simulink model "MinSeg_Controller"  (R2014b)
settings: Solver=FixedStepDiscrete  SolverMode=SingleTasking  StartTime=0.0  StopTime=inf  FixedStep=TS  RelTol=1e-3
PostLoadFcn:
  | clc
  | 
  | fprintf('Loading MinSegConfigSet...\n')
  | load('MinSegConfig');
  | 
  | fprintf('Attaching MinSegConfigSet...\n')
  | try % Will error if already attached
  | MinSegConfigSet.Name = 'MinSegConfigSet';
  | attachConfigSet('MinSeg_Controller',MinSegConfigSet,false);
  | end
  | 
  | fprintf('Activating MinSegConfigSet...\n')
  | setActiveConfigSet('MinSeg_Controller','MinSegConfigSet');
  | 
  | fprintf('Loading Parameters...\n')
  | MinSeg_Parameters;
  | 
  | fprintf('Model setup complete.\n')
values from neighbouring files (symbols this model uses):
  ES = -C2DEG*D2R    (= -0.00872664625997)    [MinSeg_Parameters.m]    (also in MinSeg_Parameters_v2.m; MinSeg_Parameters_v3.m)
  GS = GyroS*D2R    (= 0.000155832968928)    [MinSeg_Parameters.m]    (also in MinSeg_Parameters_v2.m; MinSeg_Parameters_v3.m)
  Ki = 1*[-r_w -r_w*0 1 1*0]    [MinSeg_Parameters.m]    (also in MinSeg_Parameters_v2.m; MinSeg_Parameters_v3.m)
  KLQRC = KLQR.*[-r_w -r_w 1 1]    [MinSeg_Parameters.m]    (also in MinSeg_Parameters_v2.m; MinSeg_Parameters_v3.m)
  TS = .03    (= 0.03)    [MinSeg_Parameters.m]    (also in MinSeg_Parameters_v2.m = 0.005; MinSeg_Parameters_v3.m = 0.005)
  tstart = 2    [MinSeg_Parameters.m]    (also in MinSeg_Parameters_v2.m; MinSeg_Parameters_v3.m)
  V2DCB = 1/DCB2V    (= 42.5)    [MinSeg_Parameters.m]    (also in MinSeg_Parameters_v2.m = 28.3333333333; MinSeg_Parameters_v3.m = 28.3333333333)
undefined symbols (not defined in the file or in its folder): K
libraries: simulink x4, arduinolib x3, powerlib_meascontrol x1
settings Model: SimulationMode=external  ExtModeTrigDuration=2  Creator=hrlin  LastModifiedBy=mo114c
settings OptimizationCC: ExpressionDepthLimit=2147483647  OptimizeModelRefInitCode=on  LifeSpan=1
settings DebuggingCC: UnderspecifiedInitializationDetection=Classic  MergeDetectMultiDrivingBlocksExec=none  SolverPrmCheckMsg=none  StateNameClashWarn=warning
settings HardwareCC: ProdBitPerInt=16  ProdBitPerPointer=8  ProdIntDivRoundTo=Zero  ProdEndianess=LittleEndian  ProdWordSize=8  ProdHWDeviceType=Atmel->AVR
settings RTWCC: SystemTargetFile=realtime.tlc  GenerateMakefile=off  TemplateMakefile=realtime.tmf  Description=Real-Time Toolbox  RTWVerbose=off  ProcessScript=realtime_make_rtw_hook
settings CodeAppCC: CustomSymbolStrType=$N$R$M  InternalIdentifier=Classic
settings STFCustomTargetCC: TargetLibSuffix=.a  GenerateSampleERTMain=on  ERTCustomFileBanners=on  SupportNonInlinedSFcns=off  SupportVariableSizeSignals=on  MATLABClassNameForMDSCustomization=Simulink.SoftwareTarget.ERTCustomization  GRTInterface=off  SystemTargetFile=realtime.tlc
settings ERTTargetCC: GenerateSampleERTMain=on  ParMdlRefBuildCompliant=off  CompOptLevelCompliant=off  ConcurrentExecutionCompliant=off  CombineOutputUpdateFcns=off  ERTFirstTimeCompliant=off  SupportContinuousTime=on  SupportVariableSizeSignals=on  ModelStepFunctionPrototypeControlCompliant=off  CPPClassGenCompliant=off  ExtMode=on  ExtModeTransport=3  ExtModeMexFile=ext_serial_win32_comm  ExtModeMexArgs=0 4 115200 30  InlinedParameterPlacement=NonHierarchical  ERTSrcFileBannerTemplate=realtime_code_template.cgt  ERTHdrFileBannerTemplate=realtime_code_template.cgt  ERTDataSrcFileTemplate=realtime_code_template.cgt  ERTDataHdrFileTemplate=realtime_code_template.cgt  ERTCustomFileTemplate=realtime_file_process.tlc

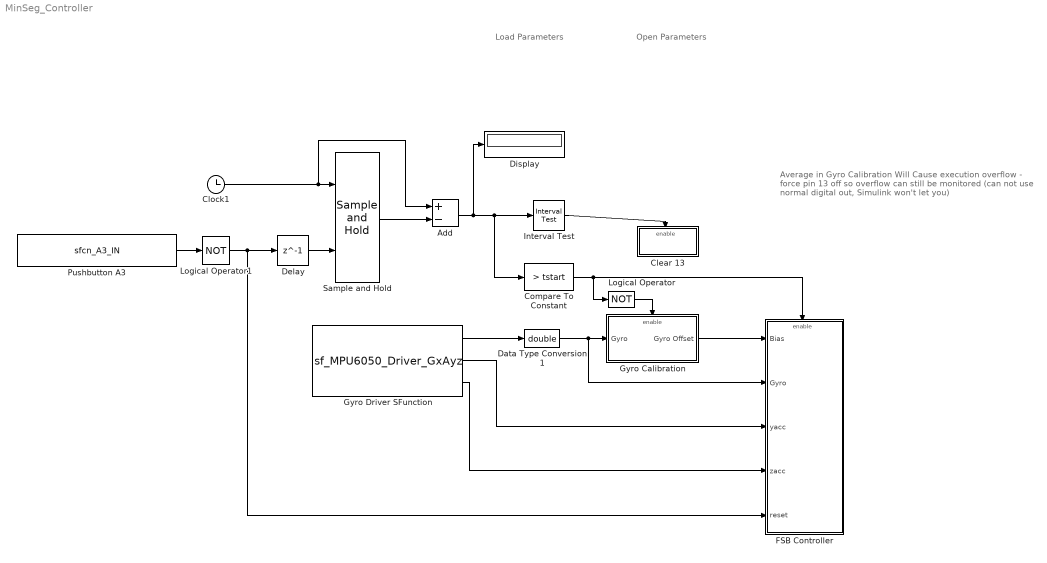
== system MinSeg_Controller ==
  note: Average in Gyro Calibration Will
      | Cause execution overflow - force pin 13 off
      | so overflow can still be monitored (can not use normal
      | digital out, Simulink won't let you)
  note: Load Parameters
  note: Open Parameters
  Add : Sum  Inputs=+-
  "Clear 13 " : Subsystem  TreatAsAtomicUnit=on
  Clock1 : Clock
  Compare To Constant : simulink/Logic and Bit Operations/Compare To Constant  relop=>  const=tstart  OutDataTypeStr=boolean
  Data Type Conversion1 : DataTypeConversion  OutDataTypeStr=double
  Delay : Delay  DelayLength=1
  Display : Display
  FSB Controller : Subsystem
  Gyro Calibration : Subsystem  TreatAsAtomicUnit=on
  Gyro Driver SFunction : S-Function  InitFcn=try, set_param(gcb,'FunctionName','sf_MPU6050_Driver_GxAyz'), end  FunctionName=sf_MPU6050_Driver_GxAyz  SFunctionModules=sf_MPU6050_Driver_GxAyz_wrapper  EnableBusSupport=off  mask(S-Function Builder){}
      mask help: Simulink:masks:SFunctionBuilder_MD
      mask init:
      | val = [[.9  0.75 0.75 1 1 .9 .9 1]',[1 1 0.75 0.75 .9 .9 1 .9]'];try , sys = get_param(gcb,'SfunBuilderFcnName');if isempty(sys), sys = get_param(gcb,'FunctionName'); end,catch, sys = get_param(gcb,'FunctionName'); end
      settings: CopyFcn=set_param(gcbh,'LinkStatus','none')  PreSaveFcn=try, set_param(gcb,'FunctionName','sf_MPU6050_Driver_GxAyz'), end  OpenFcn=sfunctionwizard(gcbh)
      mask Display: plot(val(:,1),val(:,2)),disp(sys), port_label('output',1,'x_vel'), port_label('output',2,'y_acc'), port_label('output',3,'z_acc')
  Interval Test : simulink/Logic and Bit Operations/Interval Test  IntervalClosedRight=off  uplimit=tstart+0.1  IntervalClosedLeft=off  lowlimit=tstart  OutDataTypeStr=boolean
  Logical Operator1 : Logic  Operator=NOT  AllPortsSameDT=off  OutDataTypeStr=boolean
  Logical Operator : Logic  Operator=NOT  AllPortsSameDT=off  OutDataTypeStr=boolean
  Pushbutton A3 : S-Function  InitFcn=try, set_param(gcb,'FunctionName','sfcn_A3_IN'), end  FunctionName=sfcn_A3_IN  SFunctionModules=sfcn_A3_IN_wrapper  EnableBusSupport=off  mask(S-Function Builder){}
      mask help: Simulink:masks:SFunctionBuilder_MD
      mask init: same as MinSeg_Controller/Gyro Driver SFunction
      settings: CopyFcn=set_param(gcbh,'LinkStatus','none')  PreSaveFcn=try, set_param(gcb,'FunctionName','sfcn_A3_IN'), end  OpenFcn=sfunctionwizard(gcbh)
      mask Display: plot(val(:,1),val(:,2)),disp(sys), port_label('output',1,'push_button')
  Sample and Hold : powerlib_meascontrol/Additional Components/Sample and Hold  ic=0  Ts=0
  wires:
  Compare To Constant/1 -> Logical Operator/1, FSB Controller/Enable
  Gyro Calibration/1(Gyro Offset) -> FSB Controller/1(Bias)
  Gyro Driver SFunction/1 -> Data Type Conversion1/1
  Logical Operator/1 -> Gyro Calibration/Enable
  Data Type Conversion1/1 -> FSB Controller/2(Gyro), Gyro Calibration/1(Gyro)
  Interval Test/1 -> "Clear 13 "/Enable
  Gyro Driver SFunction/2 -> FSB Controller/3("yacc ")
  Gyro Driver SFunction/3 -> FSB Controller/4("zacc ")
  Pushbutton A3/1 -> Logical Operator1/1
  Clock1/1 -> Add/1, Sample and Hold/1
  Sample and Hold/1 -> Add/2
  Add/1 -> Display/1, Compare To Constant/1, Interval Test/1
  Logical Operator1/1 -> FSB Controller/5(reset), Delay/1
  Delay/1 -> Sample and Hold/2

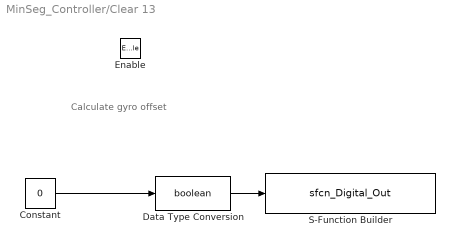
== system MinSeg_Controller/Clear 13  ==
  note: Calculate gyro offset
  Enable : EnablePort  StatesWhenEnabling=reset
  Constant : Constant  Value=0
  Data Type Conversion : DataTypeConversion  OutDataTypeStr=boolean
  S-Function Builder : S-Function  InitFcn=try, set_param(gcb,'FunctionName','sfcn_Digital_Out'), end  FunctionName=sfcn_Digital_Out  Parameters=uint8(13)  SFunctionModules=sfcn_Digital_Out_wrapper  EnableBusSupport=off  mask(S-Function Builder){}
      mask init: same as MinSeg_Controller/Gyro Driver SFunction
      settings: CopyFcn=set_param(gcbh,'LinkStatus','none')  PreSaveFcn=try, set_param(gcb,'FunctionName','sfcn_Digital_Out'), end  OpenFcn=sfunctionwizard(gcbh)
      mask Display: plot(val(:,1),val(:,2)),disp(sys), port_label('input',1,'in')
  wires:
  Data Type Conversion/1 -> S-Function Builder/1
  Constant/1 -> Data Type Conversion/1

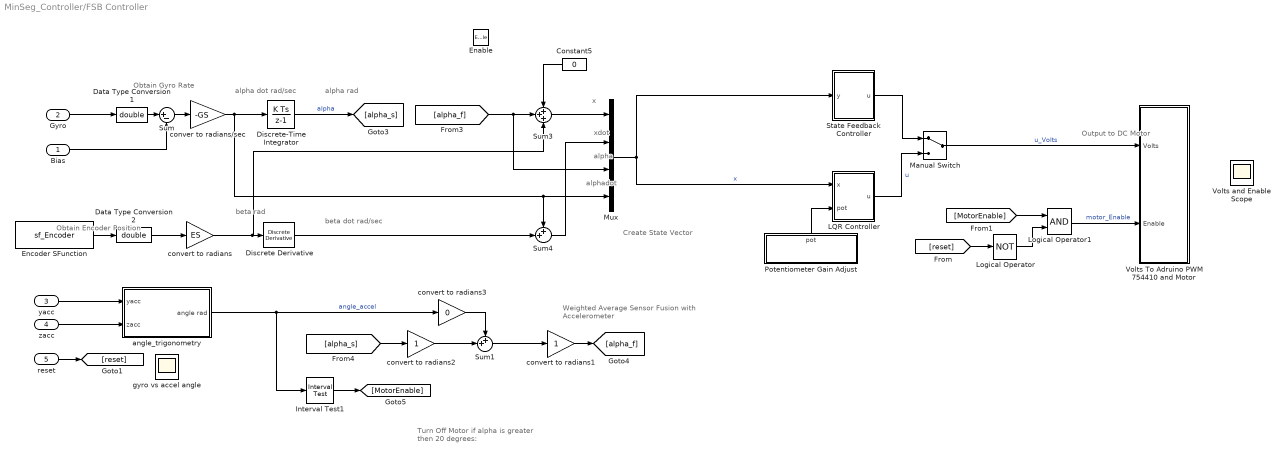
== system MinSeg_Controller/FSB Controller ==
  note: Weighted Average Sensor
      | Fusion with Accelerometer
  note: Turn Off Motor if alpha is
      | greater then 20 degrees:
  note: Output to DC Motor
  note: Create State Vector
  note: Obtain Encoder Position
  note: Obtain Gyro Rate
  note: xdot
  note: x
  note: beta
      | rad
  note: alpha dot
      | rad/sec
  note: alpha
      | rad
  note: beta dot
      | rad/sec
  note: alpha
  note: alphadot
  Bias : Inport
  Gyro : Inport  Port=2
  "yacc " : Inport  Port=3
  "zacc " : Inport  Port=4
  reset : Inport  Port=5
  Enable : EnablePort  StatesWhenEnabling=reset
  Constant5 : Constant  Value=0
  Data Type Conversion1 : DataTypeConversion  OutDataTypeStr=double
  Data Type Conversion2 : DataTypeConversion  OutDataTypeStr=double
  Discrete Derivative : simulink/Discrete/Discrete Derivative  gainval=1.0  ICPrevScaledInput=0.0  InputProcessing=Inherited  OutMin=[]  OutMax=[]  OutDataType=fixdt(1, 16)  OutScaling=2^-10  DoSatur=off
  Discrete-Time Integrator : DiscreteIntegrator  SampleTime=TS
  Encoder SFunction : S-Function  InitFcn=try, set_param(gcb,'FunctionName','sf_Encoder'), end  FunctionName=sf_Encoder  Parameters=uint8(0),uint8(18),uint8(19)  SFunctionModules=sf_Encoder_wrapper  EnableBusSupport=off  mask(S-Function Builder){}
      mask init: same as MinSeg_Controller/Gyro Driver SFunction
      settings: CopyFcn=set_param(gcbh,'LinkStatus','none')  PreSaveFcn=try, set_param(gcb,'FunctionName','sf_Encoder'), end  OpenFcn=sfunctionwizard(gcbh)
      mask Display: plot(val(:,1),val(:,2)),disp(sys), port_label('output',1,'pos')
  Interval Test1 : simulink/Logic and Bit Operations/Interval Test  IntervalClosedRight=off  uplimit=0.75  IntervalClosedLeft=off  lowlimit=-0.75  OutDataTypeStr=boolean
  LQR Controller : Subsystem
  Logical Operator : Logic  Operator=NOT  AllPortsSameDT=off  OutDataTypeStr=boolean
  Logical Operator1 : Logic  AllPortsSameDT=off  OutDataTypeStr=boolean
  Manual Switch : ManualSwitch
  Mux : Mux
  Potentiometer Gain Adjust : Subsystem
  State Feedback Controller : Subsystem
  Sum : Sum  Inputs=|+-
  Sum1 : Sum  Inputs=++|
  Sum3 : Sum  Inputs=+++
  Sum4 : Sum  Inputs=++|
  Volts To Adruino PWM 754410 and Motor : Subsystem
  Volts and Enable Scope : Scope  NumInputPorts=2
      settings: Floating=on  YMin=0~0  YMax=1~1
  angle_trigonometry : Subsystem
  conver to radians/sec : Gain  Gain=-GS
  convert to radians : Gain  Gain=ES  OutDataTypeStr=double
  convert to radians1 : Gain  OutDataTypeStr=double
  convert to radians2 : Gain  OutDataTypeStr=double
  convert to radians3 : Gain  Gain=0  OutDataTypeStr=double
  gyro vs accel angle : Scope  NumInputPorts=2
      settings: Floating=on  YMin=-0.4~-2  YMax=0.3~1.5
  wires:
  Sum3/1 -> Mux/1
  Data Type Conversion2/1 -> convert to radians/1
  Bias/1 -> Sum/2
  Sum/1 -> conver to radians/sec/1
  Encoder SFunction/1 -> Data Type Conversion2/1
  convert to radians/1 -> Discrete Derivative/1, Sum3/3
  Data Type Conversion1/1 -> Sum/1
  Gyro/1 -> Data Type Conversion1/1
  Discrete Derivative/1 -> Sum4/2
  conver to radians/sec/1 -> Discrete-Time Integrator/1, Sum4/1, Mux/4
  Sum4/1 -> Mux/2
  Discrete-Time Integrator/1 -> [alpha_s]  "alpha"
  Constant5/1 -> Sum3/1
  "yacc "/1 -> angle_trigonometry/1(yacc)
  "zacc "/1 -> angle_trigonometry/2(zacc)
  angle_trigonometry/1(angle rad) -> Interval Test1/1, convert to radians3/1  "angle_accel"
  [alpha_f] -> Mux/3, Sum3/2
  [alpha_s] -> convert to radians2/1
  Sum1/1 -> convert to radians1/1
  convert to radians1/1 -> [alpha_f]
  convert to radians2/1 -> Sum1/2
  convert to radians3/1 -> Sum1/1
  Mux/1 -> State Feedback Controller/1(y), LQR Controller/1(x)  "x"
  LQR Controller/1(u) -> Manual Switch/2  "u"
  State Feedback Controller/1(u) -> Manual Switch/1
  Manual Switch/1 -> Volts To Adruino PWM 754410 and Motor/1(Volts)  "u_Volts"
  reset/1 -> [reset]
  [reset] -> Logical Operator/1
  Logical Operator/1 -> Logical Operator1/2
  Logical Operator1/1 -> Volts To Adruino PWM 754410 and Motor/2(Enable)  "motor_Enable"
  [MotorEnable] -> Logical Operator1/1
  Potentiometer Gain Adjust/1(pot) -> LQR Controller/2(pot)
  Interval Test1/1 -> [MotorEnable]

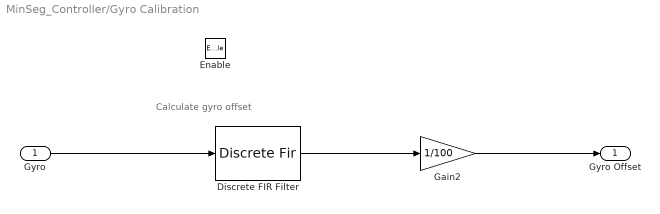
== system MinSeg_Controller/Gyro Calibration ==
  note: Calculate gyro offset
  Gyro : Inport
  Enable : EnablePort  StatesWhenEnabling=reset
  Discrete FIR Filter : DiscreteFir  Coefficients=ones(1,100)
  Gain2 : Gain  Gain=1/100  OutDataTypeStr=Inherit: Same as input  ParamDataTypeStr=Inherit: Same as input
  Gyro Offset : Outport
  wires:
  Gyro/1 -> Discrete FIR Filter/1
  Discrete FIR Filter/1 -> Gain2/1
  Gain2/1 -> Gyro Offset/1

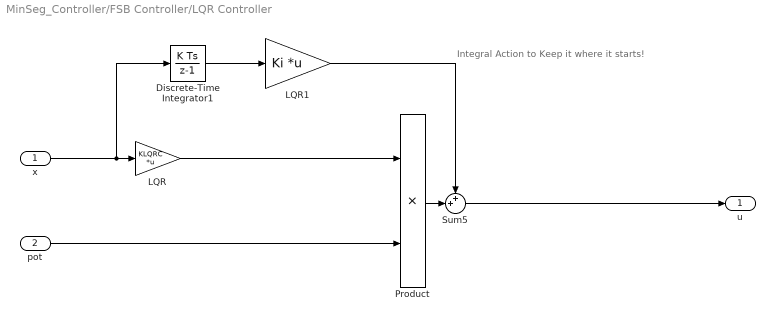
== system MinSeg_Controller/FSB Controller/LQR Controller ==
  note: Integral Action to Keep it where it starts!
  x : Inport
  pot : Inport  Port=2
  Discrete-Time Integrator1 : DiscreteIntegrator  SampleTime=TS
  LQR : Gain  Gain=KLQRC  Multiplication=Matrix(K*u)
  LQR1 : Gain  Gain=Ki  Multiplication=Matrix(K*u)
  Product : Product  RndMeth=Zero
  Sum5 : Sum  Inputs=++|
  u : Outport
  wires:
  x/1 -> Discrete-Time Integrator1/1, LQR/1
  Discrete-Time Integrator1/1 -> LQR1/1
  Product/1 -> Sum5/2
  LQR/1 -> Product/1
  LQR1/1 -> Sum5/1
  Sum5/1 -> u/1
  pot/1 -> Product/2

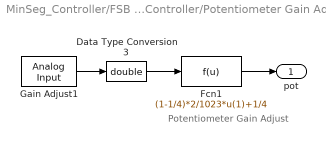
== system MinSeg_Controller/FSB Controller/Potentiometer Gain Adjust ==
  note: Potentiometer Gain Adjust
  Data Type Conversion3 : DataTypeConversion  OutDataTypeStr=double
  Fcn1 : Fcn  Expr=(1-1/4)*2/1023*u(1)+1/4
  Gain Adjust1 : arduinolib/Analog Input  pinNumber=0  sampleTime=-1  blockPlatform=arduino
  pot : Outport
  wires:
  Data Type Conversion3/1 -> Fcn1/1
  Fcn1/1 -> pot/1
  Gain Adjust1/1 -> Data Type Conversion3/1

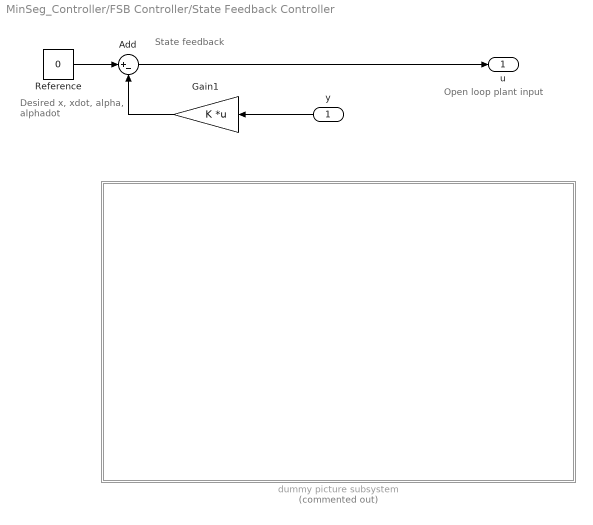
== system MinSeg_Controller/FSB Controller/State Feedback Controller ==
  note: Desired x, xdot,
      | alpha, alphadot
  note: State feedback
  note: Open loop plant input
  y : Inport
  Add : Sum  Inputs=|+-
  Gain1 : Gain  Gain=K  Multiplication=Matrix(K*u)
  Reference : Constant  Value=0
  dummy picture subsystem : Subsystem  Commented=on  TreatAsAtomicUnit=on
      settings: RTWFcnNameOpts=Use subsystem name  RTWFileNameOpts=Use function name
      mask Display: image(imread('SFBK.png'))
  u : Outport
  wires:
  Add/1 -> u/1
  Gain1/1 -> Add/2
  Reference/1 -> Add/1
  y/1 -> Gain1/1

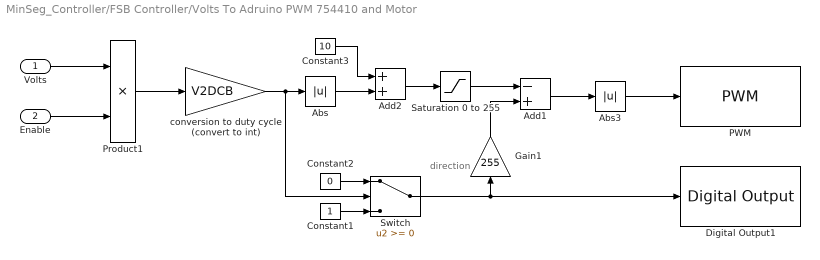
== system MinSeg_Controller/FSB Controller/Volts To Adruino PWM 754410 and Motor ==
  note: direction
  Volts : Inport
  Enable : Inport  Port=2
  Abs : Abs
  Abs3 : Abs
  Add1 : Sum  Inputs=-+
  Add2 : Sum
  Constant1 : Constant
  Constant2 : Constant  Value=0
  Constant3 : Constant  Value=10
  Digital Output1 : arduinolib/Digital Output  pinNumber=6  blockPlatform=arduino
  Gain1 : Gain  Gain=255
  PWM : arduinolib/PWM  pinNumber=8  blockPlatform=arduino
  Product1 : Product  RndMeth=Zero
  Saturation 0 to 255 : Saturate  UpperLimit=255  LowerLimit=0
  Switch : Switch
  conversion to duty cycle (convert to int) : Gain  Gain=V2DCB  OutDataTypeStr=int16
  wires:
  Volts/1 -> Product1/1
  Switch/1 -> Digital Output1/1, Gain1/1
  Constant2/1 -> Switch/1
  Constant1/1 -> Switch/3
  Gain1/1 -> Add1/2
  Add1/1 -> Abs3/1
  conversion to duty cycle (convert to int)/1 -> Switch/2, Abs/1
  Saturation 0 to 255/1 -> Add1/1
  Abs3/1 -> PWM/1
  Constant3/1 -> Add2/1
  Abs/1 -> Add2/2
  Add2/1 -> Saturation 0 to 255/1
  Enable/1 -> Product1/2
  Product1/1 -> conversion to duty cycle (convert to int)/1

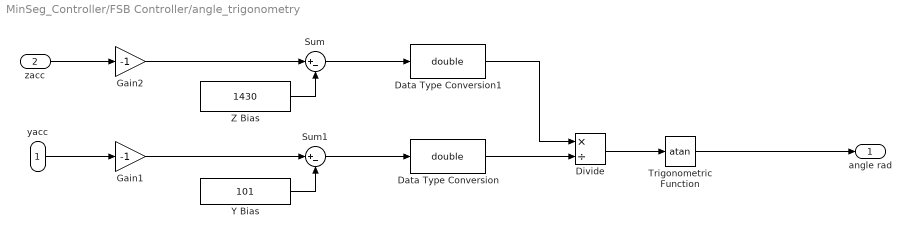
== system MinSeg_Controller/FSB Controller/angle_trigonometry ==
  yacc : Inport
  zacc : Inport  Port=2
  Data Type Conversion : DataTypeConversion  OutDataTypeStr=double
  Data Type Conversion1 : DataTypeConversion  OutDataTypeStr=double
  Divide : Product  Inputs=*/
  Gain1 : Gain  Gain=-1
  Gain2 : Gain  Gain=-1
  Sum : Sum  Inputs=|+-
  Sum1 : Sum  Inputs=|+-
  Trigonometric Function : Trigonometry  Operator=atan
  Y Bias : Constant  Value=101
  Z Bias : Constant  Value=1430
  angle rad : Outport
  wires:
  Sum1/1 -> Data Type Conversion/1
  Gain2/1 -> Sum/1
  Sum/1 -> Data Type Conversion1/1
  Z Bias/1 -> Sum/2
  Gain1/1 -> Sum1/1
  Y Bias/1 -> Sum1/2
  Trigonometric Function/1 -> angle rad/1
  Divide/1 -> Trigonometric Function/1
  zacc/1 -> Gain2/1
  yacc/1 -> Gain1/1
  Data Type Conversion1/1 -> Divide/1
  Data Type Conversion/1 -> Divide/2

== system MinSeg_Controller/FSB Controller/State Feedback Controller/dummy picture subsystem ==
